simulink model "Test_RealSwArcForUFOEn_SoftwareSystemArchitecture_mapping"  (R2016b)
settings: Solver=FixedStepAuto  StartTime=0.0  StopTime=10.0  RelTol=1e-3
model workspace: external: MAT-File Test_RealSwArcForUFOEn_SoftwareSystemArchitecture_mapping.mat (data not in the file)
libraries: libAsserts x4, libTLAsserts x4
settings Model: Creator=NEATdemo  LastModifiedBy=NEATdemo

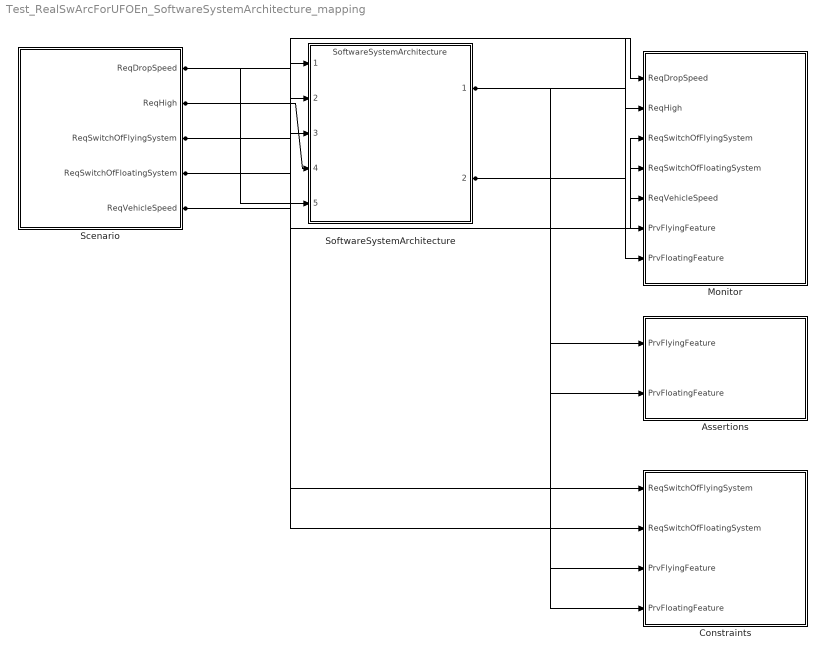
== system Test_RealSwArcForUFOEn_SoftwareSystemArchitecture_mapping ==
  Assertions : Subsystem
  Constraints : Subsystem
  Monitor : Subsystem
  Scenario : Subsystem
  SoftwareSystemArchitecture : ModelReference  ModelNameDialog=SoftwareSystemArchitecture  SimulationMode=Normal  ModelReferenceVersion=1.12
  wires:
  Scenario/1(ReqDropSpeed) -> SoftwareSystemArchitecture/5, Monitor/1(ReqDropSpeed)
  Scenario/2(ReqHigh) -> SoftwareSystemArchitecture/4, Monitor/2(ReqHigh)
  Scenario/4(ReqSwitchOfFloatingSystem) -> SoftwareSystemArchitecture/3, Monitor/4(ReqSwitchOfFloatingSystem), Constraints/2(ReqSwitchOfFloatingSystem)
  Scenario/3(ReqSwitchOfFlyingSystem) -> SoftwareSystemArchitecture/2, Monitor/3(ReqSwitchOfFlyingSystem), Constraints/1(ReqSwitchOfFlyingSystem)
  Scenario/5(ReqVehicleSpeed) -> SoftwareSystemArchitecture/1, Monitor/5(ReqVehicleSpeed)
  SoftwareSystemArchitecture/1 -> Monitor/6(PrvFlyingFeature), Assertions/1(PrvFlyingFeature), Constraints/3(PrvFlyingFeature)
  SoftwareSystemArchitecture/2 -> Monitor/7(PrvFloatingFeature), Assertions/2(PrvFloatingFeature), Constraints/4(PrvFloatingFeature)

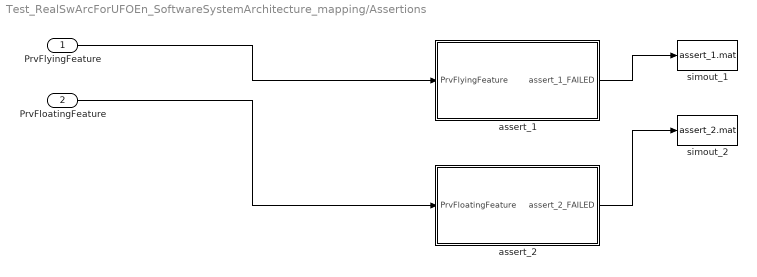
== system Test_RealSwArcForUFOEn_SoftwareSystemArchitecture_mapping/Assertions ==
  PrvFlyingFeature : Inport
  PrvFloatingFeature : Inport  Port=2
  assert_1 : Subsystem
  assert_2 : Subsystem
  simout_1 : ToFile  Filename=assert_1.mat  MatrixName=assert_1  SaveFormat=Timeseries
  simout_2 : ToFile  Filename=assert_2.mat  MatrixName=assert_2  SaveFormat=Timeseries
  wires:
  PrvFlyingFeature/1 -> assert_1/1(PrvFlyingFeature)
  assert_1/1(assert_1_FAILED) -> simout_1/1
  PrvFloatingFeature/1 -> assert_2/1(PrvFloatingFeature)
  assert_2/1(assert_2_FAILED) -> simout_2/1

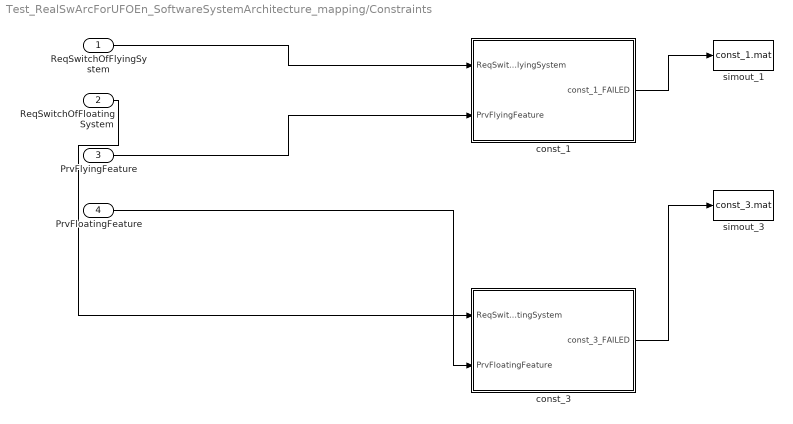
== system Test_RealSwArcForUFOEn_SoftwareSystemArchitecture_mapping/Constraints ==
  ReqSwitchOfFlyingSystem : Inport
  ReqSwitchOfFloatingSystem : Inport  Port=2
  PrvFlyingFeature : Inport  Port=3
  PrvFloatingFeature : Inport  Port=4
  const_1 : Subsystem
  const_3 : Subsystem
  simout_1 : ToFile  Filename=const_1.mat  MatrixName=const_1  SaveFormat=Timeseries
  simout_3 : ToFile  Filename=const_3.mat  MatrixName=const_3  SaveFormat=Timeseries
  wires:
  ReqSwitchOfFlyingSystem/1 -> const_1/1(ReqSwitchOfFlyingSystem)
  PrvFlyingFeature/1 -> const_1/2(PrvFlyingFeature)
  const_1/1(const_1_FAILED) -> simout_1/1
  ReqSwitchOfFloatingSystem/1 -> const_3/1(ReqSwitchOfFloatingSystem)
  PrvFloatingFeature/1 -> const_3/2(PrvFloatingFeature)
  const_3/1(const_3_FAILED) -> simout_3/1

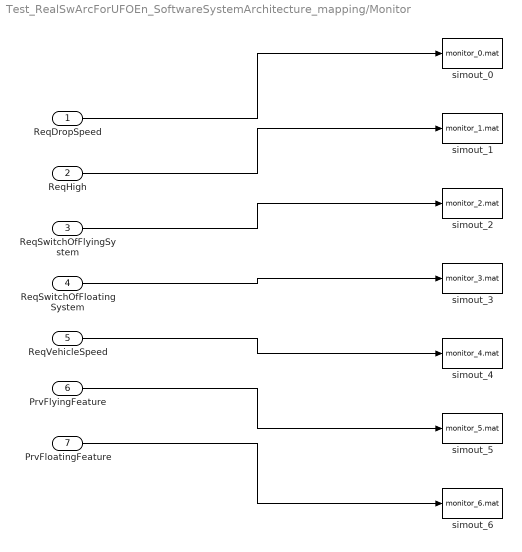
== system Test_RealSwArcForUFOEn_SoftwareSystemArchitecture_mapping/Monitor ==
  ReqDropSpeed : Inport
  ReqHigh : Inport  Port=2
  ReqSwitchOfFlyingSystem : Inport  Port=3
  ReqSwitchOfFloatingSystem : Inport  Port=4
  ReqVehicleSpeed : Inport  Port=5
  PrvFlyingFeature : Inport  Port=6
  PrvFloatingFeature : Inport  Port=7
  simout_0 : ToFile  Filename=monitor_0.mat  MatrixName=ReqDropSpeed  SaveFormat=Timeseries
  simout_1 : ToFile  Filename=monitor_1.mat  MatrixName=ReqHigh  SaveFormat=Timeseries
  simout_2 : ToFile  Filename=monitor_2.mat  MatrixName=ReqSwitchOfFlyingSystem  SaveFormat=Timeseries
  simout_3 : ToFile  Filename=monitor_3.mat  MatrixName=ReqSwitchOfFloatingSystem  SaveFormat=Timeseries
  simout_4 : ToFile  Filename=monitor_4.mat  MatrixName=ReqVehicleSpeed  SaveFormat=Timeseries
  simout_5 : ToFile  Filename=monitor_5.mat  MatrixName=PrvFlyingFeature  SaveFormat=Timeseries
  simout_6 : ToFile  Filename=monitor_6.mat  MatrixName=PrvFloatingFeature  SaveFormat=Timeseries
  wires:
  ReqDropSpeed/1 -> simout_0/1
  ReqHigh/1 -> simout_1/1
  ReqSwitchOfFlyingSystem/1 -> simout_2/1
  ReqSwitchOfFloatingSystem/1 -> simout_3/1
  ReqVehicleSpeed/1 -> simout_4/1
  PrvFlyingFeature/1 -> simout_5/1
  PrvFloatingFeature/1 -> simout_6/1

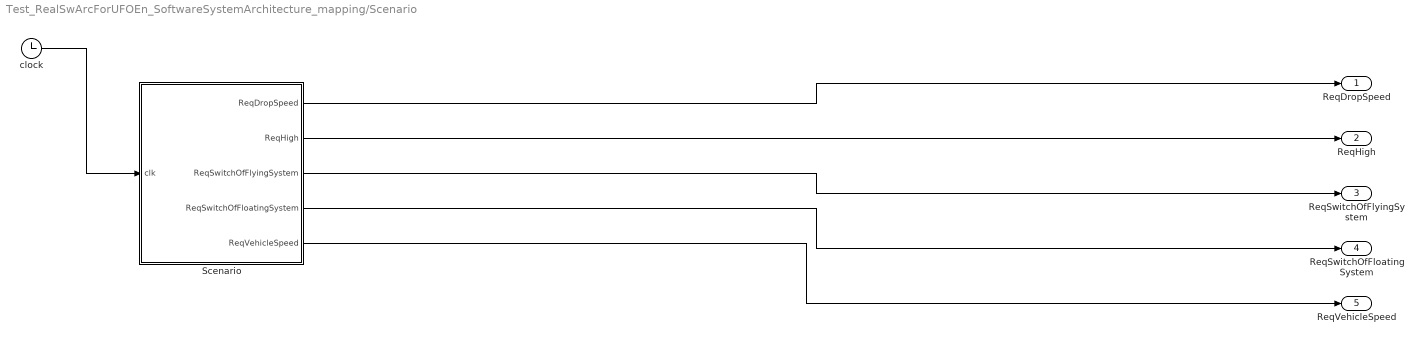
== system Test_RealSwArcForUFOEn_SoftwareSystemArchitecture_mapping/Scenario ==
  Scenario : Stateflow chart  TreatAsAtomicUnit=on
  clock : Clock
  ReqDropSpeed : Outport
  ReqHigh : Outport  Port=2
  ReqSwitchOfFlyingSystem : Outport  Port=3
  ReqSwitchOfFloatingSystem : Outport  Port=4
  ReqVehicleSpeed : Outport  Port=5
  wires:
  Scenario/1(ReqDropSpeed) -> ReqDropSpeed/1
  Scenario/2(ReqHigh) -> ReqHigh/1
  Scenario/4(ReqSwitchOfFloatingSystem) -> ReqSwitchOfFloatingSystem/1
  Scenario/3(ReqSwitchOfFlyingSystem) -> ReqSwitchOfFlyingSystem/1
  Scenario/5(ReqVehicleSpeed) -> ReqVehicleSpeed/1
  clock/1 -> Scenario/1(clk)

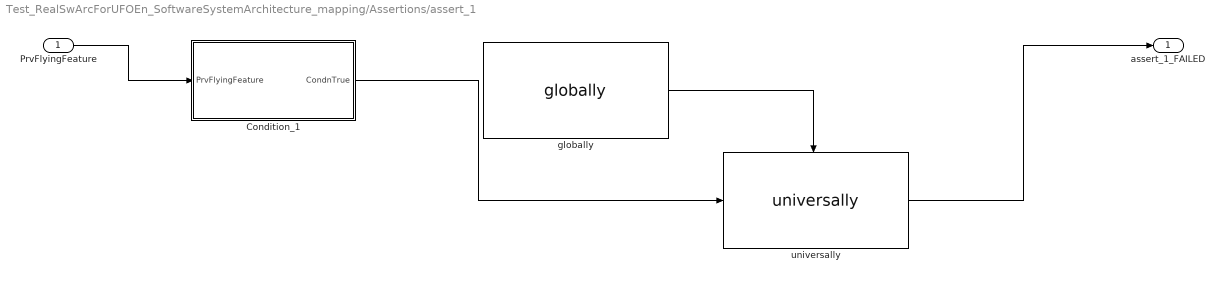
== system Test_RealSwArcForUFOEn_SoftwareSystemArchitecture_mapping/Assertions/assert_1 ==
  PrvFlyingFeature : Inport
  Condition_1 : Subsystem
  globally : libAsserts/globally
  universally : libAsserts/universally
  assert_1_FAILED : Outport
  wires:
  PrvFlyingFeature/1 -> Condition_1/1(PrvFlyingFeature)
  Condition_1/1(CondnTrue) -> universally/1
  universally/1 -> assert_1_FAILED/1
  globally/1 -> universally/Enable

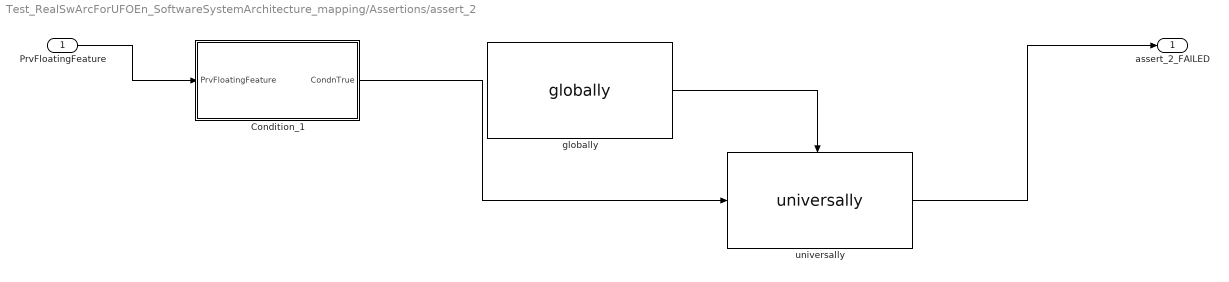
== system Test_RealSwArcForUFOEn_SoftwareSystemArchitecture_mapping/Assertions/assert_2 ==
  PrvFloatingFeature : Inport
  Condition_1 : Subsystem
  globally : libAsserts/globally
  universally : libAsserts/universally
  assert_2_FAILED : Outport
  wires:
  PrvFloatingFeature/1 -> Condition_1/1(PrvFloatingFeature)
  Condition_1/1(CondnTrue) -> universally/1
  universally/1 -> assert_2_FAILED/1
  globally/1 -> universally/Enable

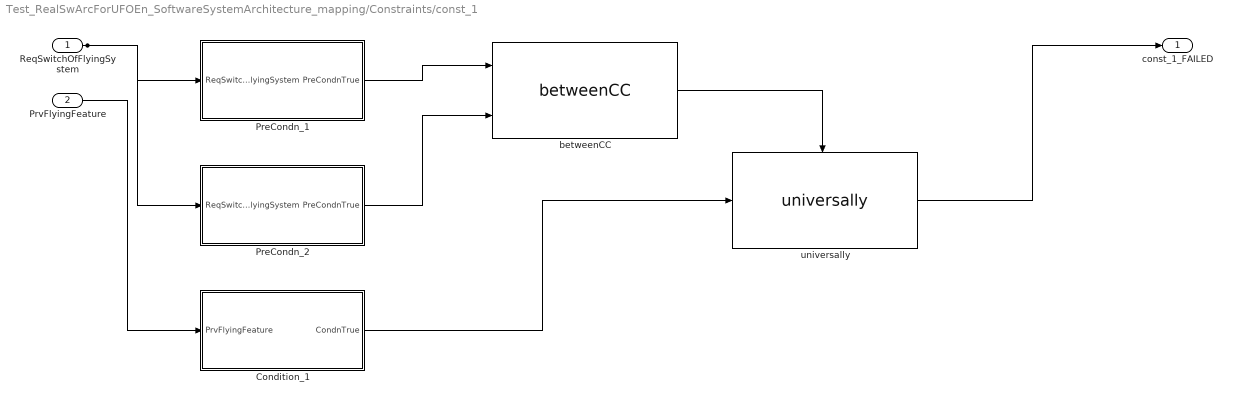
== system Test_RealSwArcForUFOEn_SoftwareSystemArchitecture_mapping/Constraints/const_1 ==
  ReqSwitchOfFlyingSystem : Inport
  PrvFlyingFeature : Inport  Port=2
  Condition_1 : Subsystem
  PreCondn_1 : Subsystem
  PreCondn_2 : Subsystem
  betweenCC : libTLAsserts/betweenCC
  universally : libTLAsserts/universally
  const_1_FAILED : Outport
  wires:
  ReqSwitchOfFlyingSystem/1 -> PreCondn_1/1(ReqSwitchOfFlyingSystem), PreCondn_2/1(ReqSwitchOfFlyingSystem)
  PrvFlyingFeature/1 -> Condition_1/1(PrvFlyingFeature)
  PreCondn_1/1(PreCondnTrue) -> betweenCC/1
  PreCondn_2/1(PreCondnTrue) -> betweenCC/2
  Condition_1/1(CondnTrue) -> universally/1
  betweenCC/1 -> universally/Enable
  universally/1 -> const_1_FAILED/1

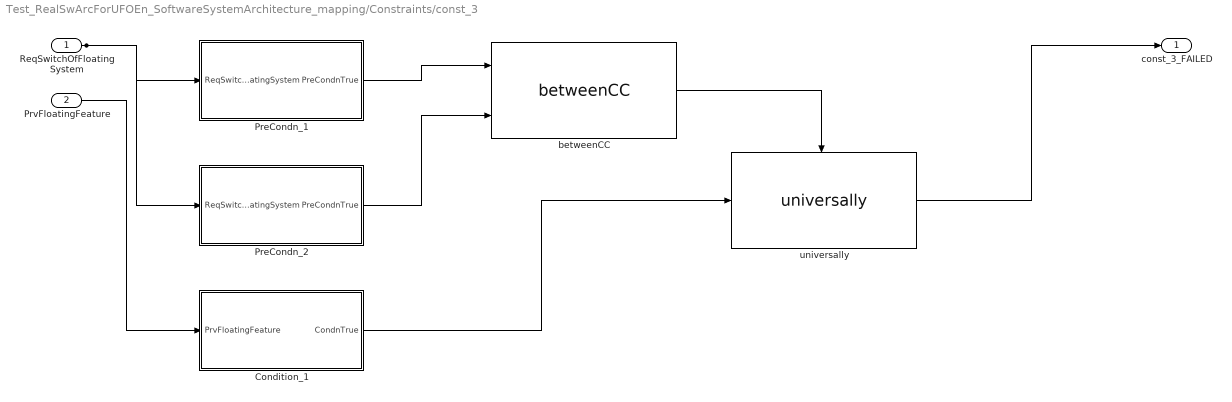
== system Test_RealSwArcForUFOEn_SoftwareSystemArchitecture_mapping/Constraints/const_3 ==
  ReqSwitchOfFloatingSystem : Inport
  PrvFloatingFeature : Inport  Port=2
  Condition_1 : Subsystem
  PreCondn_1 : Subsystem
  PreCondn_2 : Subsystem
  betweenCC : libTLAsserts/betweenCC
  universally : libTLAsserts/universally
  const_3_FAILED : Outport
  wires:
  ReqSwitchOfFloatingSystem/1 -> PreCondn_1/1(ReqSwitchOfFloatingSystem), PreCondn_2/1(ReqSwitchOfFloatingSystem)
  PrvFloatingFeature/1 -> Condition_1/1(PrvFloatingFeature)
  PreCondn_1/1(PreCondnTrue) -> betweenCC/1
  PreCondn_2/1(PreCondnTrue) -> betweenCC/2
  Condition_1/1(CondnTrue) -> universally/1
  betweenCC/1 -> universally/Enable
  universally/1 -> const_3_FAILED/1

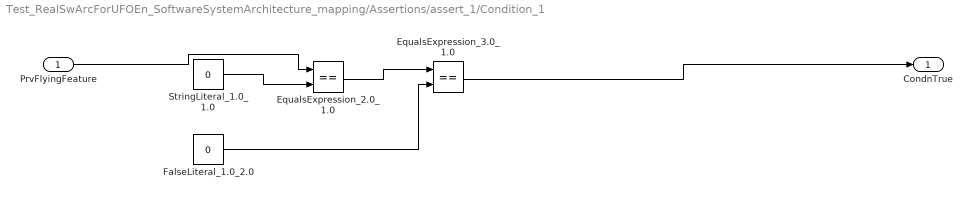
== system Test_RealSwArcForUFOEn_SoftwareSystemArchitecture_mapping/Assertions/assert_1/Condition_1 ==
  PrvFlyingFeature : Inport
  EqualsExpression_2.0_1.0 : RelationalOperator  Operator===  OutDataTypeStr=boolean  RndMeth=Simplest
  EqualsExpression_3.0_1.0 : RelationalOperator  Operator===  OutDataTypeStr=boolean  RndMeth=Simplest
  FalseLiteral_1.0_2.0 : Constant  Value=0
  StringLiteral_1.0_1.0 : Constant  Value=0
  CondnTrue : Outport
  wires:
  PrvFlyingFeature/1 -> EqualsExpression_2.0_1.0/1
  StringLiteral_1.0_1.0/1 -> EqualsExpression_2.0_1.0/2
  EqualsExpression_2.0_1.0/1 -> EqualsExpression_3.0_1.0/1
  FalseLiteral_1.0_2.0/1 -> EqualsExpression_3.0_1.0/2
  EqualsExpression_3.0_1.0/1 -> CondnTrue/1

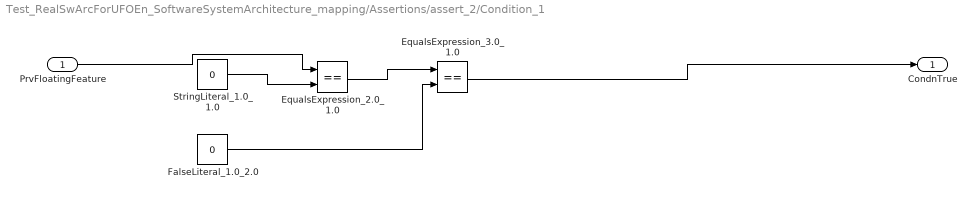
== system Test_RealSwArcForUFOEn_SoftwareSystemArchitecture_mapping/Assertions/assert_2/Condition_1 ==
  PrvFloatingFeature : Inport
  EqualsExpression_2.0_1.0 : RelationalOperator  Operator===  OutDataTypeStr=boolean  RndMeth=Simplest
  EqualsExpression_3.0_1.0 : RelationalOperator  Operator===  OutDataTypeStr=boolean  RndMeth=Simplest
  FalseLiteral_1.0_2.0 : Constant  Value=0
  StringLiteral_1.0_1.0 : Constant  Value=0
  CondnTrue : Outport
  wires:
  PrvFloatingFeature/1 -> EqualsExpression_2.0_1.0/1
  StringLiteral_1.0_1.0/1 -> EqualsExpression_2.0_1.0/2
  EqualsExpression_2.0_1.0/1 -> EqualsExpression_3.0_1.0/1
  FalseLiteral_1.0_2.0/1 -> EqualsExpression_3.0_1.0/2
  EqualsExpression_3.0_1.0/1 -> CondnTrue/1

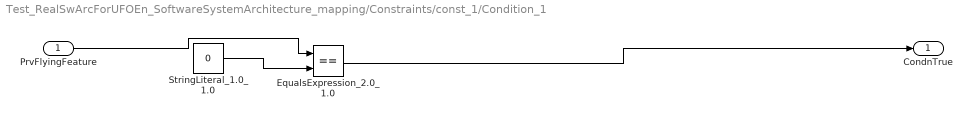
== system Test_RealSwArcForUFOEn_SoftwareSystemArchitecture_mapping/Constraints/const_1/Condition_1 ==
  PrvFlyingFeature : Inport
  EqualsExpression_2.0_1.0 : RelationalOperator  Operator===  OutDataTypeStr=boolean  RndMeth=Simplest
  StringLiteral_1.0_1.0 : Constant  Value=0
  CondnTrue : Outport
  wires:
  PrvFlyingFeature/1 -> EqualsExpression_2.0_1.0/1
  StringLiteral_1.0_1.0/1 -> EqualsExpression_2.0_1.0/2
  EqualsExpression_2.0_1.0/1 -> CondnTrue/1

== system Test_RealSwArcForUFOEn_SoftwareSystemArchitecture_mapping/Constraints/const_1/PreCondn_1 ==
  ReqSwitchOfFlyingSystem : Inport
  PreCondnTrue : Outport
  wires:
  ReqSwitchOfFlyingSystem/1 -> PreCondnTrue/1

== system Test_RealSwArcForUFOEn_SoftwareSystemArchitecture_mapping/Constraints/const_1/PreCondn_2 ==
  ReqSwitchOfFlyingSystem : Inport
  EqualsExpression_2.0_1.0 : RelationalOperator  Operator===  OutDataTypeStr=boolean  RndMeth=Simplest
  FalseLiteral_1.0_1.0 : Constant  Value=0
  PreCondnTrue : Outport
  wires:
  ReqSwitchOfFlyingSystem/1 -> EqualsExpression_2.0_1.0/1
  FalseLiteral_1.0_1.0/1 -> EqualsExpression_2.0_1.0/2
  EqualsExpression_2.0_1.0/1 -> PreCondnTrue/1

== system Test_RealSwArcForUFOEn_SoftwareSystemArchitecture_mapping/Constraints/const_3/Condition_1 ==
  PrvFloatingFeature : Inport
  EqualsExpression_2.0_1.0 : RelationalOperator  Operator===  OutDataTypeStr=boolean  RndMeth=Simplest
  StringLiteral_1.0_1.0 : Constant  Value=0
  CondnTrue : Outport
  wires:
  PrvFloatingFeature/1 -> EqualsExpression_2.0_1.0/1
  StringLiteral_1.0_1.0/1 -> EqualsExpression_2.0_1.0/2
  EqualsExpression_2.0_1.0/1 -> CondnTrue/1

== system Test_RealSwArcForUFOEn_SoftwareSystemArchitecture_mapping/Constraints/const_3/PreCondn_1 ==
  ReqSwitchOfFloatingSystem : Inport
  PreCondnTrue : Outport
  wires:
  ReqSwitchOfFloatingSystem/1 -> PreCondnTrue/1

== system Test_RealSwArcForUFOEn_SoftwareSystemArchitecture_mapping/Constraints/const_3/PreCondn_2 ==
  ReqSwitchOfFloatingSystem : Inport
  EqualsExpression_2.0_1.0 : RelationalOperator  Operator===  OutDataTypeStr=boolean  RndMeth=Simplest
  FalseLiteral_1.0_1.0 : Constant  Value=0
  PreCondnTrue : Outport
  wires:
  ReqSwitchOfFloatingSystem/1 -> EqualsExpression_2.0_1.0/1
  FalseLiteral_1.0_1.0/1 -> EqualsExpression_2.0_1.0/2
  EqualsExpression_2.0_1.0/1 -> PreCondnTrue/1

== stateflow chart Test_RealSwArcForUFOEn_SoftwareSystemArchitecture_mapping/Scenario/Scenario ==
  state Act_Car_Step1
    entry: ReqDropSpeed = 0;
    entry: ReqHigh = 0;
    entry: ReqSwitchOfFloatingSystem = 0;
    entry: ReqSwitchOfFlyingSystem = 0;
    entry: ReqVehicleSpeed = 0;
  state Act_Car_Step2
    entry: ReqVehicleSpeed = ReqVehicleSpeed + 1;
    entry: Act_Car_Step2_stpClk = clk;
  state Act_Car_Step3
    entry: ReqSwitchOfFlyingSystem = 1;
  state Act_Car_Step4
    entry: Act_Car_Step4_stpClk = clk;
  (default) -> Act_Car_Step1
  Act_Car_Step1 -> Act_Car_Step2
  Act_Car_Step2 -> Act_Car_Step3 : [clk - Act_Car_Step2_stpClk >= 10]
  Act_Car_Step3 -> Act_Car_Step4
  data: clk input; ReqDropSpeed output; ReqHigh output; ReqSwitchOfFlyingSystem output; ReqSwitchOfFloatingSystem output; ReqVehicleSpeed output; Act_Car_Step2_stpClk local; Act_Car_Step4_stpClk local
